simulink model "leaderSineVel"  (R2018b)
settings: Solver=VariableStepAuto  StartTime=0.0  StopTime=inf  RelTol=1e-3
undefined symbols (not defined in the file or in its folder): Angular, Linear
libraries: robotlib x2
settings Model: Creator=ckreienk  LastModifiedBy=ckreienk

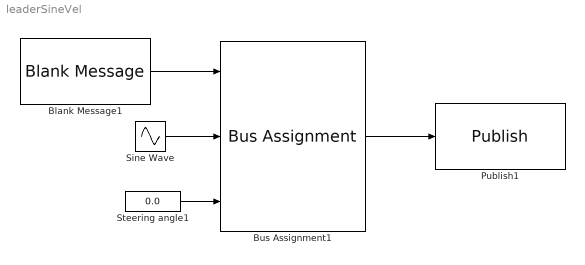
== system leaderSineVel ==
  Blank Message1 : robotlib/Blank Message  messageClass=Message  entityType=geometry_msgs/Twist  messageType=geometry_msgs/Twist  SampleTime=inf
      settings: SourceProductBaseCode=RO
  Bus Assignment1 : BusAssignment  AssignedSignals=Linear.X,Angular.Z
  Publish1 : robotlib/Publish  topicSource=Select from ROS network  topic=/leadVehicle/cmd_vel  messageType=geometry_msgs/Twist  messageQueueLength=1
      settings: SourceProductBaseCode=RO
  Sine Wave : Sin  Amplitude=4  Bias=3  Frequency=3  SampleTime=0
  Steering angle1 : Constant  Value=0.0
  wires:
  Bus Assignment1/1 -> Publish1/1
  Blank Message1/1 -> Bus Assignment1/1
  Sine Wave/1 -> Bus Assignment1/2
  Steering angle1/1 -> Bus Assignment1/3
